simulink model "ShowerSystem"  (R2024a)
settings: Solver=VariableStepAuto  StartTime=0.0  StopTime=10.0  RelTol=1e-3
settings Model: Creator=Admin  LastModifiedBy=Admin

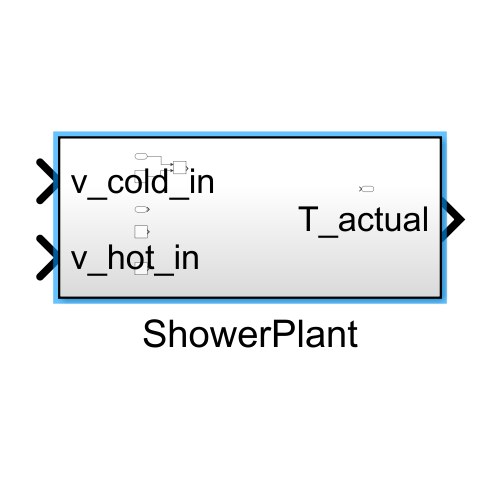
[thumbnail: Simulink's stored preview of the top-level diagram]
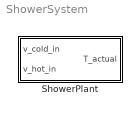
== system ShowerSystem ==
  ShowerPlant : Subsystem

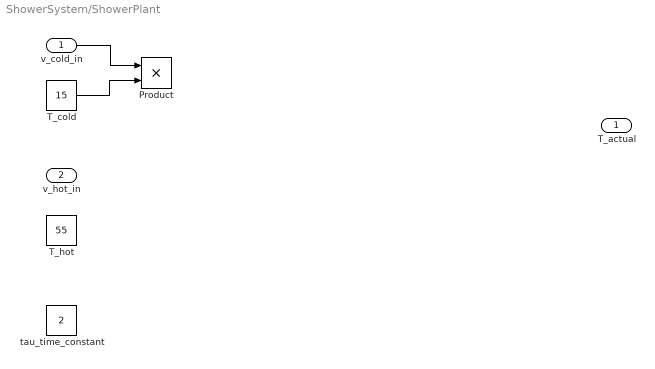
== system ShowerSystem/ShowerPlant ==
  v_cold_in : Inport
  v_hot_in : Inport  Port=2
  Product : Product
  T_cold : Constant  Value=15
  T_hot : Constant  Value=55
  tau_time_constant : Constant  Value=2
  T_actual : Outport
  wires:
  v_cold_in/1 -> Product/1
  T_cold/1 -> Product/2
